simulink model "sim_lab5_zadanie2"  (R2023b)
settings: Solver=FixedStepAuto  StartTime=0.0  StopTime=200  FixedStep=0.001  RelTol=1e-3
values from neighbouring files (symbols this model uses):
  disc_model = c2d( cont_model, Ts )    [laboratorium5.m]    (also in zadanie2.m)
  final_value = 1    [Copy_of_zadanie2.m]    (also in laboratorium5.m; zadanie2.m)
  init_value = 0    [Copy_of_zadanie2.m]    (also in laboratorium5.m; zadanie2.m)
  pi_disc_model = c2d ( pi_cont_model, Ts2 )    [zadanie2.m]
  time_step = 0    [Copy_of_zadanie2.m]    (also in laboratorium5.m; zadanie2.m)
  Ts = 0.5    [laboratorium5.m]    (also in zadanie2.m = 0.001)
  Ts2 = Ts_Control_Vector(j)    [zadanie2.m]
settings Model: Creator=student  LastModifiedBy=tomasz
settings SolverCC: AlgebraicLoopSolver=TrustRegion
settings DebuggingCC: UnconnectedInputMsg=warning  UnconnectedOutputMsg=warning  UnconnectedLineMsg=warning
settings ModelReferenceCC: EnableRefExpFcnMdlSchedulingChecks=on
settings RTWCC: DLArmComputeVersion=19.05

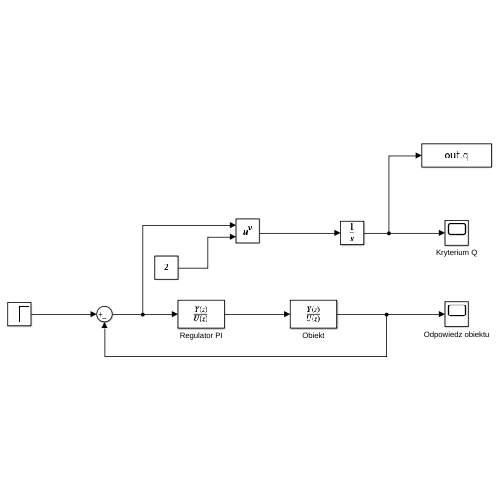
[thumbnail: Simulink's stored preview of the top-level diagram]
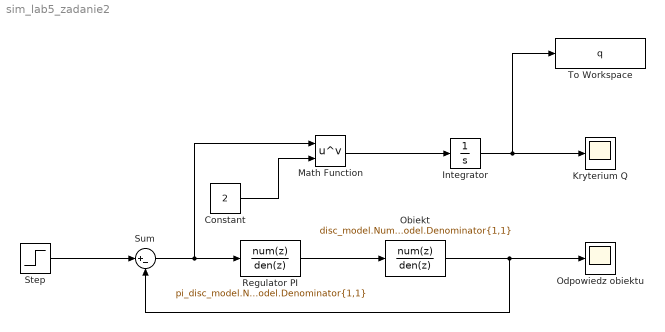
== system sim_lab5_zadanie2 ==
  Constant : Constant  Value=2
  Integrator : Integrator
  Kryterium Q : Scope
  Math Function : Math  Operator=pow
  Obiekt : DiscreteTransferFcn  Numerator=disc_model.Numerator{1,1}  Denominator=disc_model.Denominator{1,1}  SampleTime=Ts
  Odpowiedz obiektu : Scope
  Regulator PI : DiscreteTransferFcn  Numerator=pi_disc_model.Numerator{1,1}  Denominator=pi_disc_model.Denominator{1,1}  SampleTime=Ts2
  Step : Step  Time=time_step  Before=init_value  After=final_value  SampleTime=0
  Sum : Sum  Inputs=|+-
  To Workspace : ToWorkspace  VariableName=q  SaveFormat=Timeseries  SampleTime=-1
  wires:
  Step/1 -> Sum/1
  Sum/1 -> Math Function/1, Regulator PI/1
  Regulator PI/1 -> Obiekt/1
  Obiekt/1 -> Sum/2, Odpowiedz obiektu/1
  Math Function/1 -> Integrator/1
  Integrator/1 -> To Workspace/1, Kryterium Q/1
  Constant/1 -> Math Function/2
